simulink model "SUB_IoControl"  (R2018b)
(part 6 of 8)

  Data Type Conversion14/1 -> out_OUT_PCAN.Tx_Out.Out_11_Sts.Out_STATUS/1
  Data Type Conversion15/1 -> out_OUT_PCAN.Tx_Out.Out_16_Sts.Out_STATUS/1
  Data Type Conversion16/1 -> out_OUT_PCAN.Tx_Out.Out_17_Sts.Out_STATUS/1
  Data Type Conversion18/1 -> out_OUT_PCAN.Tx_Out.Out_19_Sts.Out_STATUS/1
  in_IN_DigitalOutputsSTATIC.OUT_01_SENSE_PULSE/1 -> out_OUT_PCAN.Tx_Out.Out_01_TD_Sts.Out_SENSE_PULSE/1
  in_DIAG_DigitalOutputsSTATIC.OUT_01_SENSE_PULSE_DIAG/1 -> out_OUT_PCAN.Tx_Out.Out_01_TD_Sts.Out_SENSE_PULSE_DIAG/1
  in_IN_DigitalOutputsSTATIC.OUT_04_SENSE_PULSE/1 -> out_OUT_PCAN.Tx_Out.Out_04_TD_Sts.Out_SENSE_PULSE/1
  in_DIAG_DigitalOutputsSTATIC.OUT_04_SENSE_PULSE_DIAG/1 -> out_OUT_PCAN.Tx_Out.Out_04_TD_Sts.Out_SENSE_PULSE_DIAG/1
  in_IN_DigitalOutputsSTATIC.OUT_07_SENSE_PULSE/1 -> out_OUT_PCAN.Tx_Out.Out_07_TD_Sts.Out_SENSE_PULSE/1
  in_DIAG_DigitalOutputsSTATIC.OUT_07_SENSE_PULSE_DIAG/1 -> out_OUT_PCAN.Tx_Out.Out_07_TD_Sts.Out_SENSE_PULSE_DIAG/1
  in_IN_DigitalOutputsSTATIC.OUT_06_SENSE_PULSE/1 -> out_OUT_PCAN.Tx_Out.Out_06_TD_Sts.Out_SENSE_PULSE/1
  in_DIAG_DigitalOutputsSTATIC.OUT_06_SENSE_PULSE_DIAG/1 -> out_OUT_PCAN.Tx_Out.Out_06_TD_Sts.Out_SENSE_PULSE_DIAG/1
  in_IN_DigitalOutputsSTATIC.OUT_08_SENSE_PULSE/1 -> out_OUT_PCAN.Tx_Out.Out_08_TD_Sts.Out_SENSE_PULSE/1
  in_DIAG_DigitalOutputsSTATIC.OUT_08_SENSE_PULSE_DIAG/1 -> out_OUT_PCAN.Tx_Out.Out_08_TD_Sts.Out_SENSE_PULSE_DIAG/1
  in_IN_DigitalOutputsSTATIC.OUT_12_SENSE_PULSE/1 -> out_OUT_PCAN.Tx_Out.Out_12_TD_Sts.Out_SENSE_PULSE/1
  in_DIAG_DigitalOutputsSTATIC.OUT_12_SENSE_PULSE_DIAG/1 -> out_OUT_PCAN.Tx_Out.Out_12_TD_Sts.Out_SENSE_PULSE_DIAG/1
  in_IN_DigitalOutputsSTATIC.OUT_13_SENSE_PULSE/1 -> out_OUT_PCAN.Tx_Out.Out_13_TD_Sts.Out_SENSE_PULSE/1
  in_DIAG_DigitalOutputsSTATIC.OUT_13_SENSE_PULSE_DIAG/1 -> out_OUT_PCAN.Tx_Out.Out_13_TD_Sts.Out_SENSE_PULSE_DIAG/1
  in_IN_DigitalOutputsSTATIC.OUT_14_SENSE_PULSE/1 -> out_OUT_PCAN.Tx_Out.Out_14_TD_Sts.Out_SENSE_PULSE/1
  in_DIAG_DigitalOutputsSTATIC.OUT_14_SENSE_PULSE_DIAG/1 -> out_OUT_PCAN.Tx_Out.Out_14_TD_Sts.Out_SENSE_PULSE_DIAG/1
  in_IN_DigitalOutputsSTATIC.OUT_15_SENSE_PULSE/1 -> out_OUT_PCAN.Tx_Out.Out_15_TD_Sts.Out_SENSE_PULSE/1
  in_DIAG_DigitalOutputsSTATIC.OUT_15_SENSE_PULSE_DIAG/1 -> out_OUT_PCAN.Tx_Out.Out_15_TD_Sts.Out_SENSE_PULSE_DIAG/1
  in_IN_PCAN.Rx_Ctrl.Out_Ctrl.Out_03_Ctrl/1 -> MOD_OutputDiag_Ctrl_03/1
  in_IN_PCAN.Rx_Ctrl.Out_Ctrl.Out_05_Ctrl/1 -> MOD_OutputDiag_Ctrl_05/1
  in_IN_PCAN.Rx_Ctrl.Out_Ctrl.Out_09_Ctrl/1 -> MOD_OutputDiag_Ctrl_09/1
  in_IN_PCAN.Rx_Ctrl.Out_Ctrl.Out_10_Ctrl/1 -> MOD_OutputDiag_Ctrl_10/1
  in_IN_PCAN.Rx_Ctrl.Out_Ctrl.Out_11_Ctrl/1 -> MOD_OutputDiag_Ctrl_11/1
  in_IN_PCAN.Rx_Ctrl.Out_Ctrl.Out_16_Ctrl/1 -> MOD_OutputDiag_Ctrl_16/1
  in_IN_PCAN.Rx_Ctrl.Out_Ctrl.Out_17_Ctrl/1 -> MOD_OutputDiag_Ctrl_17/1
  in_IN_PCAN.Rx_Ctrl.Out_Ctrl.Out_19_Ctrl/1 -> MOD_OutputDiag_Ctrl_19/1
  MOD_TrailerDetection_Ctrl_01/1 -> MOD_OutputDiag_Ctrl_01/1
  [boCtrlValid] -> MOD_OutputDiag_Ctrl_15/3, MOD_OutputDiag_Ctrl_14/3, MOD_OutputDiag_Ctrl_13/3, MOD_OutputDiag_Ctrl_12/3, MOD_OutputDiag_Ctrl_08/3, MOD_OutputDiag_Ctrl_07/3, MOD_OutputDiag_Ctrl_06/3, MOD_OutputDiag_Ctrl_04/3, MOD_OutputDiag_Ctrl_01/3
  MOD_TrailerDetection_Ctrl_04/1 -> MOD_OutputDiag_Ctrl_04/1
  MOD_TrailerDetection_Ctrl_06/1 -> MOD_OutputDiag_Ctrl_06/1
  MOD_TrailerDetection_Ctrl_07/1 -> MOD_OutputDiag_Ctrl_07/1
  MOD_TrailerDetection_Ctrl_08/1 -> MOD_OutputDiag_Ctrl_08/1
  MOD_TrailerDetection_Ctrl_12/1 -> MOD_OutputDiag_Ctrl_12/1
  MOD_TrailerDetection_Ctrl_13/1 -> MOD_OutputDiag_Ctrl_13/1
  MOD_TrailerDetection_Ctrl_14/1 -> MOD_OutputDiag_Ctrl_14/1
  MOD_TrailerDetection_Ctrl_15/1 -> MOD_OutputDiag_Ctrl_15/1
  [boOut_02_DIAG] -> MOD_OutputDiag_Ctrl_02/2
  [boOut_03_DIAG] -> MOD_OutputDiag_Ctrl_03/2
  [boOut_05_DIAG] -> MOD_OutputDiag_Ctrl_05/2
  [boOut_09_DIAG] -> MOD_OutputDiag_Ctrl_09/2
  [boOut_10_DIAG] -> MOD_OutputDiag_Ctrl_10/2
  [boOut_11_DIAG] -> MOD_OutputDiag_Ctrl_11/2
  [boOut_16_DIAG] -> MOD_OutputDiag_Ctrl_16/2
  [boOut_17_DIAG] -> MOD_OutputDiag_Ctrl_17/2
  [boOut_19_DIAG] -> MOD_OutputDiag_Ctrl_19/2
  [boOut_01_DIAG] -> MOD_OutputDiag_Ctrl_01/2
  [boOut_04_DIAG] -> MOD_OutputDiag_Ctrl_04/2
  [boOut_06_DIAG] -> MOD_OutputDiag_Ctrl_06/2
  [boOut_07_DIAG] -> MOD_OutputDiag_Ctrl_07/2
  [boOut_08_DIAG] -> MOD_OutputDiag_Ctrl_08/2
  [boOut_12_DIAG] -> MOD_OutputDiag_Ctrl_12/2
  [boOut_13_DIAG] -> MOD_OutputDiag_Ctrl_13/2
  [boOut_14_DIAG] -> MOD_OutputDiag_Ctrl_14/2
  [boOut_15_DIAG] -> MOD_OutputDiag_Ctrl_15/2
  [boCtrlValid] -> AND1/1(u1)
  in_IN_PCAN.Rx_Ctrl.Out_Ctrl.WorkingMode/1 -> AND1/2(u2)
  AND1/1(y) -> [WorkingMode]
  [WorkingMode] -> Switch/2
  [BlinkSource] -> Switch/1
  Switch/1 -> AND10/2(u2)
  [WorkingMode] -> Switch1/2
  in_IN_PCAN.Rx_Ctrl.Out_Ctrl.Out_04_Ctrl/1 -> Switch1/3
  [BlinkSource] -> Switch1/1
  [BlinkSource] -> Switch2/1
  [WorkingMode] -> Switch2/2
  in_IN_PCAN.Rx_Ctrl.Out_Ctrl.Out_06_Ctrl/1 -> Switch2/3
  [WorkingMode] -> Switch3/2
  [BlinkSource] -> Switch3/1
  in_IN_PCAN.Rx_Ctrl.Out_Ctrl.Out_07_Ctrl/1 -> Switch3/3
  [BlinkSource] -> Switch4/1
  [WorkingMode] -> Switch4/2
  in_IN_PCAN.Rx_Ctrl.Out_Ctrl.Out_08_Ctrl/1 -> Switch4/3
  [WorkingMode] -> Switch5/2
  [BlinkSource] -> Switch5/1
  in_IN_PCAN.Rx_Ctrl.Out_Ctrl.Out_12_Ctrl/1 -> Switch5/3
  [BlinkSource] -> Switch6/1
  [WorkingMode] -> Switch6/2
  in_IN_PCAN.Rx_Ctrl.Out_Ctrl.Out_13_Ctrl/1 -> Switch6/3
  [WorkingMode] -> Switch7/2
  [BlinkSource] -> Switch7/1
  in_IN_PCAN.Rx_Ctrl.Out_Ctrl.Out_14_Ctrl/1 -> Switch7/3
  [BlinkSource] -> Switch8/1
  [WorkingMode] -> Switch8/2
  in_IN_PCAN.Rx_Ctrl.Out_Ctrl.Out_15_Ctrl/1 -> Switch8/3
  BlinkSource/1(bo_Blink) -> [BlinkSource]
  in_IN_NVM.Parameter.BlinkSourcePeriod/1 -> BlinkSource/1(u16_PeriodTime)
